simulink model "SG__MDL_IO135_setup"  (R2022b)
settings: Solver=FixedStepAuto  StartTime=0.0  StopTime=Inf  RelTol=1e-3  EnableMultiTasking=on
model workspace (MAT data in the model file):
  N = Simulink.Parameter
  N.Value = 32
  N.Description = 'Number of samples'
  N.DataType = 'auto'
  N.Complexity = 'real'
  N.Dimensions = [1 1]
  enable_source = Simulink.Parameter
  enable_source.Value = 0
  enable_source.DataType = 'boolean'
  enable_source.Complexity = 'real'
  enable_source.Dimensions = [1 1]
  ff = Simulink.Parameter
  ff.Value = 1200
  ff.DataType = 'auto'
  ff.Complexity = 'real'
  ff.Dimensions = [1 1]
  fi = Simulink.Parameter
  fi.Value = 150
  fi.DataType = 'auto'
  fi.Complexity = 'real'
  fi.Dimensions = [1 1]
  in_select = Simulink.Parameter
  in_select.Value = [1 2 3 4]
  in_select.DataType = 'auto'
  in_select.Complexity = 'real'
  in_select.Dimensions = [1 4]
  out_select = Simulink.Parameter
  out_select.Value = 1
  out_select.DataType = 'auto'
  out_select.Complexity = 'real'
  out_select.Dimensions = [1 1]
  rec = Simulink.Parameter
  rec.Value = 0
  rec.DataType = 'boolean'
  rec.Complexity = 'real'
  rec.Dimensions = [1 1]
  sweep_gain = Simulink.Parameter
  sweep_gain.Value = 0
  sweep_gain.DataType = 'auto'
  sweep_gain.Complexity = 'real'
  sweep_gain.Dimensions = [1 1]
  tmax = Simulink.Parameter
  tmax.Value = 40
  tmax.DataType = 'auto'
  tmax.Complexity = 'real'
  tmax.Dimensions = [1 1]
libraries: dspsigops x4, simulink x4, speedgoatlib_IO135 x3, hdlsllib x2, slrealtimeloglib x1, dspsrcs4 x1
settings Model: SimulationMode=external  Creator=padlewsk  LastModifiedBy=padlewsk
settings SolverCC: ConcurrentTasks=on  AlgebraicLoopSolver=TrustRegion  PositivePriorityOrder=on  AutoInsertRateTranBlk=on
settings DataIOCC: SaveFormat=StructureWithTime
settings OptimizationCC: BlockReduction=off  OptimizeBlockIOStorage=off
settings DebuggingCC: TasksWithSamePriorityMsg=none  UnconnectedInputMsg=warning  UnconnectedOutputMsg=warning  UnconnectedLineMsg=warning
settings HardwareCC: ProdBitPerLong=64  ProdLongLongMode=on  ProdHWDeviceType=Intel->x86-64 (Linux 64)
settings ModelReferenceCC: EnableRefExpFcnMdlSchedulingChecks=on
settings RTWCC: Description=Simulink Real-Time  SystemTargetFile=slrealtime.tlc  TemplateMakefile=slrealtime_default_tmf  Toolchain=Simulink Real-Time Toolchain  BuildConfiguration=Faster Runs  CodeExecutionProfiling=on  TargetLang=C++

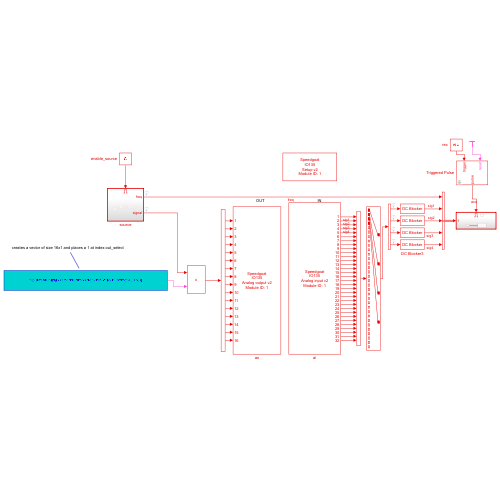
[thumbnail: Simulink's stored preview of the top-level diagram]
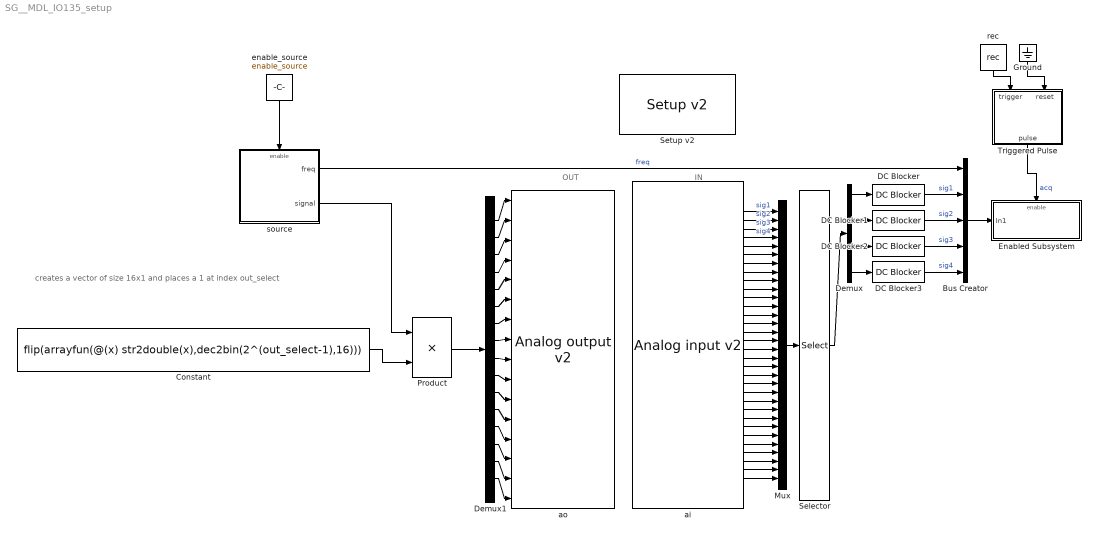
== system SG__MDL_IO135_setup ==
  note: creates a vector of size 16x1 and places a 1 at index out_select
  note: IN
  note: OUT
  Bus Creator : BusCreator  Inputs=5
  Constant : Constant  Value=flip(arrayfun(@(x) str2double(x),dec2bin(2^(out_select-1),16)))
  DC Blocker{,1..3} (4 alike) : dspsigops/DC Blocker  Algorithm=IIR  NormalizedBandwidth=0.001  Length=50  Order=6  SimulateUsing=Code generation
      settings: LibrarySourceBlock=dsphdlsupportsigops/DC Blocker
  Demux : Demux
  Demux1 : Demux  Outputs=16
  Enabled Subsystem : Subsystem  TreatAsAtomicUnit=on
  Ground : Ground
  Mux : Mux  Inputs=32
  Product : Product
  Selector : Selector  InputPortWidth=32  IndexOptions=Index vector (dialog)  Indices=in_select  OutputSizes=1
  "Setup v2 " : speedgoatlib_IO135/Setup v2   parPciSlot=-1  parModuleId=1  parInterModuleSync=None  parConvClockBaseRate=20MHz  parConvClock1Divider=20000  parConvClock2Divider=20000  parFrameTriggerEnable=off  parFrameTriggerDivider=10  parConvClock1BaseRate=1  parConvClock2BaseRate=1  parFrameTriggerClock=1  parAdcChannels=[1:32]  parAdcRange1=+-5V  parAdcRange2=+-5V  parAdcRange3=+-5V  parAdcRange4=+-5V  parAdcVoltageRange=[1 1 1 1]  parAdcOversampling1=None  parAdcOversampling2=None  parAdcOversampling3=None  parAdcOversampling4=None  parAdcOversamplRate=[1 1 1 1]  parAdcAutoCorrection=on  parAdcContSampling=off  parAdcDmaEnable=off  parAdcDmaClock=Clock 1  parAdcFrameSize_=100  parAdcSampleTime_=-1  parAdcActiveDmaDevices=[1 1 1 1]  parAdcFrameTriggerEnable=0  parAdcFrameSize=100  parAdcSampleTime=0.1  parDacChannels=1:16  parDacInitValues=0  parDacReset=1  parDacRange1=+-5V  parDacRange2=+-5V  parDacRange3=+-5V  parDacRange4=+-5V  parDacRange5=+-5V  parDacRange6=+-5V  parDacRange7=+-5V  parDacRange8=+-5V  parDacRange9=+-5V  parDacRange10=+-5V  parDacRange11=0-5V  parDacRange12=+-5V  parDacRange13=+-5V  parDacRange14=+-5V  parDacRange15=+-5V  parDacRange16=+-5V  parDacVoltageRange=[4 4 4 4 4 4 4 4 4 4 1 4 4 4 4 4]  parDacAutoCorrection=on  parDacSyncOut=on  parDacDmaEnable=off  parDacDmaLatency=Until next frame  parDacDmaClock=Clock 1  parDacFrameSize_=100  parDacSampleTime_=-1  parDacActiveDmaDevices=[1 1 1 1]  parDacFrameTriggerEnable=0  parDacFrameSize=100  parDacSampleTime=0.1  parDoChannels=[1 2]  parDoInitValues=0  parDoReset=1  parDiChannels=[3 4]  parDiDebounceEnable=off  parDiDebounceTime=0  parDiDebounceValue=0  parDioPullRefFront=Pull-up 3.3V  parDioPullRefRear=Floating
      settings: SourceProductName=Simulink Real-Time: Speedgoat I/O Blockset
  Triggered Pulse : Subsystem  mask(Triggered Pulse){N=N}
      mask prompts: N "Length (N samples)"
      mask help: Generates a single pulse of N samples length
  ai : speedgoatlib_IO135/Analog input v2   parModuleId=1  parSampleTime=0.0001  parPciSlot=-1  parAdcChannels=[1 2 3 4 5 6 7 8 9 10 11 12 13 14 15 16 17 18 19 20 21 22 23 24 25 26 27 28 29 30 31 32]  parAdcVoltageRange=[1 1 1 1]  parAdcOversamplRate=[1 1 1 1]  parAdcContSampling=0  parAdcDmaEnable=0  parAdcActiveDmaDevices=[1 1 1 1]  parAdcFrameSize=100
      settings: SourceProductName=Simulink Real-Time: Speedgoat I/O Blockset
  ao : speedgoatlib_IO135/Analog output v2   parModuleId=1  parSampleTime=0.0001  parPciSlot=-1  parDacChannels=[1 2 3 4 5 6 7 8 9 10 11 12 13 14 15 16]  parDacVoltageRange=[4 4 4 4 4 4 4 4 4 4 1 4 4 4 4 4]  parDacInitValues=[0 0 0 0 0 0 0 0 0 0 0 0 0 0 0 0]  parDacReset=[1 1 1 1 1 1 1 1 1 1 1 1 1 1 1 1]  parDacSyncOut=1  parDacDmaEnable=0  parDacActiveDmaDevices=[1 1 1 1]  parDacDmaLatency=2  parDacFrameSize=100
      settings: SourceProductName=Simulink Real-Time: Speedgoat I/O Blockset
  enable_source : Constant  Value=enable_source  SampleTime=-1
  rec : Constant  Value=rec  SampleTime=-1
  source : Subsystem  TreatAsAtomicUnit=on
  wires:
  enable_source/1 -> source/Enable
  Triggered Pulse/1(pulse) -> Enabled Subsystem/Enable  "acq"
  Ground/1 -> Triggered Pulse/2(reset)
  rec/1 -> Triggered Pulse/1(trigger)
  Bus Creator/1 -> Enabled Subsystem/1(In1)
  source/1(freq) -> Bus Creator/1  "freq"
  DC Blocker/1 -> Bus Creator/2  "sig1"
  DC Blocker1/1 -> Bus Creator/3  "sig2"
  DC Blocker2/1 -> Bus Creator/4  "sig3"
  DC Blocker3/1 -> Bus Creator/5  "sig4"
  ai/1 -> Mux/1  "sig1"
  ai/2 -> Mux/2  "sig2"
  ai/3 -> Mux/3  "sig3"
  ai/4 -> Mux/4  "sig4"
  ai/5 -> Mux/5
  ai/6 -> Mux/6
  ai/7 -> Mux/7
  ai/8 -> Mux/8
  ai/9 -> Mux/9
  ai/10 -> Mux/10
  ai/11 -> Mux/11
  ai/12 -> Mux/12
  ai/13 -> Mux/13
  ai/14 -> Mux/14
  ai/15 -> Mux/15
  ai/16 -> Mux/16
  ai/17 -> Mux/17
  ai/18 -> Mux/18
  ai/19 -> Mux/19
  ai/20 -> Mux/20
  ai/21 -> Mux/21
  ai/22 -> Mux/22
  ai/23 -> Mux/23
  ai/24 -> Mux/24
  ai/25 -> Mux/25
  ai/26 -> Mux/26
  ai/27 -> Mux/27
  ai/28 -> Mux/28
  ai/29 -> Mux/29
  ai/30 -> Mux/30
  ai/31 -> Mux/31
  ai/32 -> Mux/32
  Mux/1 -> Selector/1
  Demux/1 -> DC Blocker/1
  Demux/2 -> DC Blocker1/1
  Demux/3 -> DC Blocker2/1
  Demux/4 -> DC Blocker3/1
  Selector/1 -> Demux/1
  source/2(signal) -> Product/1
  Constant/1 -> Product/2
  Demux1/1 -> ao/1
  Demux1/2 -> ao/2
  Demux1/3 -> ao/3
  Demux1/4 -> ao/4
  Demux1/5 -> ao/5
  Demux1/6 -> ao/6
  Demux1/7 -> ao/7
  Demux1/8 -> ao/8
  Demux1/9 -> ao/9
  Demux1/10 -> ao/10
  Demux1/11 -> ao/11
  Demux1/12 -> ao/12
  Demux1/13 -> ao/13
  Demux1/14 -> ao/14
  Demux1/15 -> ao/15
  Demux1/16 -> ao/16
  Product/1 -> Demux1/1

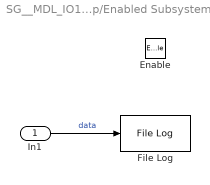
== system SG__MDL_IO135_setup/Enabled Subsystem ==
  In1 : Inport
  Enable : EnablePort
  File Log : slrealtimeloglib/File Log  decimation=1  inputProcessing=Elements as channels (sample based)
  wires:
  In1/1 -> File Log/1  "data"

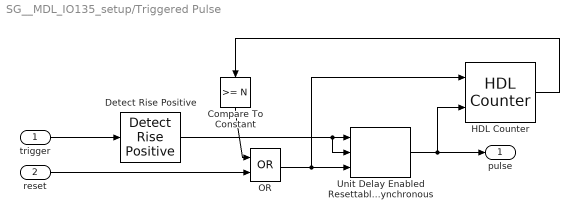
== system SG__MDL_IO135_setup/Triggered Pulse ==
  trigger : Inport
  reset : Inport  Port=2
  Compare To Constant : simulink/Logic and Bit Operations/Compare To Constant  relop=>=  const=N  OutDataTypeStr=boolean
  Detect Rise Positive : simulink/Logic and Bit Operations/Detect Rise Positive  vinit=0  OutDataTypeStr=boolean
  HDL Counter : hdlsllib/Sources/HDL Counter  CountType=Free running  CountInit=1  CountStep=1  CountMax=25  CountFromType=Initial value  CountFrom=1  CountResetPort=on  CountLoadPort=off  CountEnbPort=on  CountDirPort=off  CountHitOutputPort=off  CountDataType=Unsigned  CountWordLen=32  CountFracLen=0  CountSampTime=1
  OR : Logic  Operator=OR  AllPortsSameDT=off  OutDataTypeStr=boolean
  Unit Delay Enabled Resettable Synchronous : hdlsllib/Discrete/Unit Delay Enabled Resettable Synchronous  InitialCondition=0.0  SampleTime=-1
  pulse : Outport  VectorParamsAs1DForOutWhenUnconnected=off
  wires:
  OR/1 -> Unit Delay Enabled Resettable Synchronous/3, HDL Counter/1
  trigger/1 -> Detect Rise Positive/1
  Unit Delay Enabled Resettable Synchronous/1 -> HDL Counter/2, pulse/1
  Compare To Constant/1 -> OR/1
  reset/1 -> OR/2
  Detect Rise Positive/1 -> Unit Delay Enabled Resettable Synchronous/1, Unit Delay Enabled Resettable Synchronous/2
  HDL Counter/1 -> Compare To Constant/1

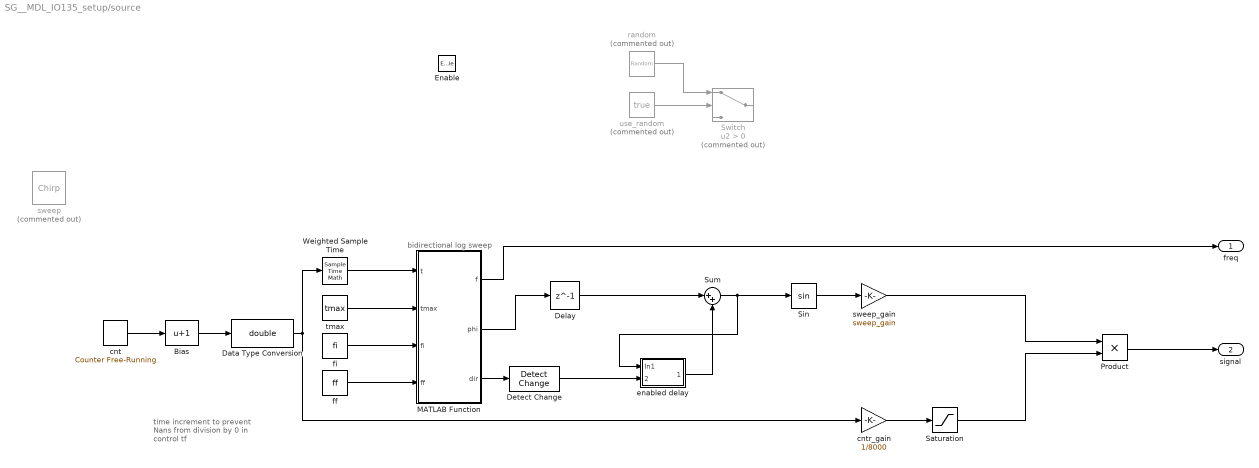
== system SG__MDL_IO135_setup/source ==
  note: bidirectional log sweep
  note: time increment to prevent Nans from division by 0 in control tf
  Enable : EnablePort  StatesWhenEnabling=reset
  Bias : Bias  Bias=1  SaturateOnIntegerOverflow=off
  Data Type Conversion : DataTypeConversion  OutDataTypeStr=double  SaturateOnIntegerOverflow=off  RndMeth=Floor
  Delay : Delay  DelayLength=1
  Detect Change : simulink/Logic and Bit Operations/Detect Change  vinit=false  OutDataTypeStr=boolean
  MATLAB Function : MATLAB Function  TreatAsAtomicUnit=on
  Product : Product
  Saturation : Saturate  UpperLimit=1  LowerLimit=0
  Sin : Trigonometry
  Sum : Sum  Inputs=|++
  Switch : Switch  Commented=on  Criteria=u2 > Threshold  SaturateOnIntegerOverflow=off  InputSameDT=off
  Weighted Sample Time : SampleTimeMath  TsampMathOp=*
  cnt : simulink/Sources/Counter Free-Running  NumBits=32  tsamp=-1
  cntr_gain : Gain  Gain=1/8000  ParamDataTypeStr=double
  enabled delay : Subsystem
  ff : Constant  Value=ff
  fi : Constant  Value=fi  VectorParams1D=off
  random : RandomNumber  Commented=on  Variance=0.5  SampleTime=3.5e-05
  sweep : dspsrcs4/Chirp  Commented=on  sweep=Logarithmic  mode=Bidirectional  f0=150  f1=1200  t1=10  Tsweep=20  phase=0  Ts=3.5e-05  spf=1  datatype=Double  OutputFrames=off
  sweep_gain : Gain  Gain=sweep_gain
  tmax : Constant  Value=tmax
  use_random : Constant  Commented=on  Value=true  SampleTime=-1
  freq : Outport  OutputWhenDisabled=reset  InitialOutput=0  VectorParamsAs1DForOutWhenUnconnected=off
  signal : Outport  Port=2  OutputWhenDisabled=reset  InitialOutput=0  VectorParamsAs1DForOutWhenUnconnected=off
  wires:
  use_random/1 -> Switch/2
  random/1 -> Switch/1
  sweep_gain/1 -> Product/1
  cntr_gain/1 -> Saturation/1
  Product/1 -> signal/1
  MATLAB Function/2(phi) -> Delay/1
  Saturation/1 -> Product/2
  Weighted Sample Time/1 -> MATLAB Function/1(t)
  Data Type Conversion/1 -> cntr_gain/1, Weighted Sample Time/1
  MATLAB Function/1(f) -> freq/1
  Sin/1 -> sweep_gain/1
  MATLAB Function/3(dir) -> Detect Change/1
  Detect Change/1 -> enabled delay/2(enable)
  Delay/1 -> Sum/1
  enabled delay/1(Out1) -> Sum/2
  Sum/1 -> enabled delay/1(In1), Sin/1
  cnt/1 -> Bias/1
  Bias/1 -> Data Type Conversion/1
  ff/1 -> MATLAB Function/4(ff)
  tmax/1 -> MATLAB Function/2(tmax)
  fi/1 -> MATLAB Function/3(fi)

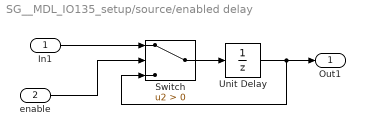
== system SG__MDL_IO135_setup/source/enabled delay ==
  In1 : Inport
  enable : Inport  Port=2
  Switch : Switch  Criteria=u2 > Threshold  SaturateOnIntegerOverflow=off  InputSameDT=off
  Unit Delay : UnitDelay  SampleTime=-1  HasFrameUpgradeWarning=on
  Out1 : Outport
  wires:
  Unit Delay/1 -> Switch/3, Out1/1
  Switch/1 -> Unit Delay/1
  In1/1 -> Switch/1
  enable/1 -> Switch/2

== matlab function SG__MDL_IO135_setup/source/MATLAB Function ==
  data: f output; t input; tmax input; phi output; dir output; fi input; ff input
function [f, phi, dir] = fcn(t, tmax, fi, ff)
%tmax is the time at which the maximum frequency is reached

t = mod(t, 2*tmax);

if t < tmax
    % up
    dir = 1;
    
    
    % linear (CF wikipedia)
%     phi = 2*pi*(0.5*(ff - fi)*t^2/tmax + fi*t);
%     f = fi + (ff - fi)*t/tmax;
    
    % logarithmic %%% https://en.wikipedia.org/wiki/Chirp
    k = log((ff/fi)^(1/tmax));
    phi = 2*pi*fi*(exp(k*t) - 1)/k;
    f = fi*exp(k*t);
else
    % down
    dir = -1;
    
    
    % linear (CF wikipedia)
%     phi = 2*pi*(0.5*(fi - ff)*(t-tmax)^2/tmax + ff*(t-tmax)); % linear
%     f = ff + (fi - ff)*(t - tmax)/tmax;
    
    % logarithmic
    k = log((fi/ff)^(1/tmax));
    phi = 2*pi*ff*(exp(k*(t - tmax)) - 1)/k;
    f = ff*exp(k*(t-tmax));
end

phi = mod(phi, 2*pi);
